simulink model "vhs_fpga_rx_sdram_8k_13xCIC"  (Simulink 7.1)
settings: Solver=FixedStepDiscrete  SolverMode=SingleTasking  StartTime=0.0  StopTime=inf  RelTol=1e-3
undefined symbols (not defined in the file or in its folder): ADC, ADCCIC, ADCClock, BasebandCIC, DAC, Fs, N_frame, N_recv_overlength, VHS
libraries: xbsIndex_r4 x230, vhsadac_common_ob_fpgalib_v1_2_0 x15, misc_tools_fpgalib_v1_0_0 x3, rapid_channel_fpgalib_v1_1_0 x2, misc_tools_dsplib_v1_0_0 x1, sdram_record_playback_fpgalib_v1_0_0 x1, rffe_fpgalib_v1_1_0 x1
(part 1 of 5)
settings Model: Creator=Administrator  LastModifiedBy=lyrtech

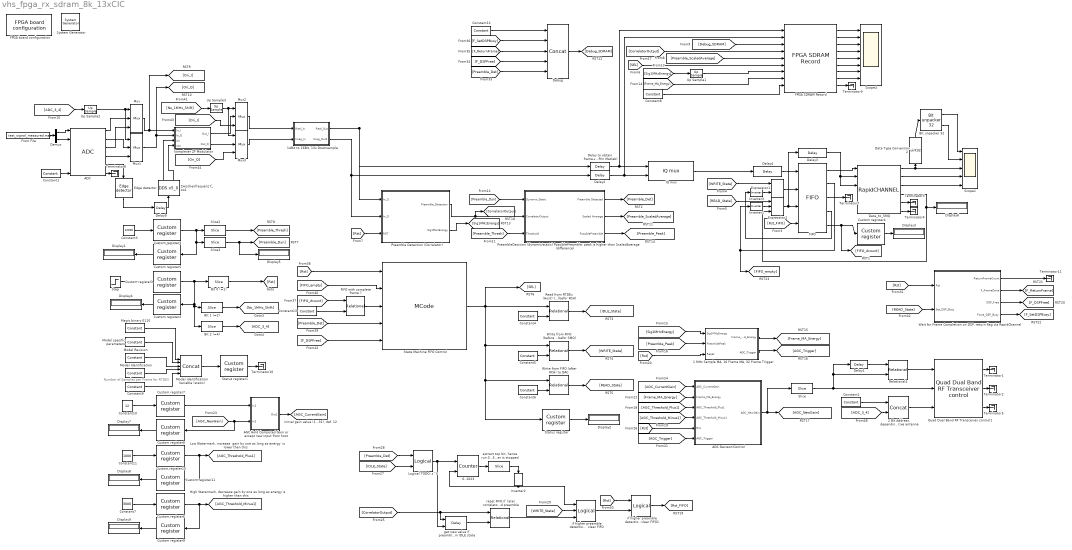
== system vhs_fpga_rx_sdram_8k_13xCIC ==
  note: Number of Samples per Frame for RTDEX
  " System Generator" : xbsIndex_r4/ System Generator  Tag=genX  SystemSampleTime=-1  xilinxfamily=virtex4  part=xc4vsx55  speed=-10  package=ff1148  synthesis_tool=XST  clock_wrapper=Clock Enables  directory=./netlist  testbench=off  simulink_period=1  sysclk_period=9  dcm_input_clock_period=100  incr_netlist=off  trim_vbits=Everywhere in SubSystem  dbl_ovrd=According to Block Masks  core_generation=According to Block Masks  run_coregen=off  deprecated_control=off  eval_field=0  block_type=sysgen
      settings: block_version=10.1.3
  0..1023 : xbsIndex_r4/Counter  cnt_type=Free Running  cnt_to=Inf  operation=Up  start_count=0  cnt_by_val=1  arith_type=Unsigned  n_bits=10  bin_pt=0  load_pin=off  rst=on  en=on  explicit_period=off  period=1  dbl_ovrd=off  use_behavioral_HDL=off  use_rpm=off  implementation=Fabric  block_type=counter
  "1 MHz Sample MA, 16 Frame MA, 32 Frame Trigger" : Subsystem
  "14Bit to 16Bit, 13x Downsample" : Subsystem
  "2 Bit Address, depending on active antenna" : xbsIndex_r4/Concat  num_inputs=2  dbl_ovrd=off  block_type=concat
      settings: block_version=10.1.3
  ADC : vhsadac_common_ob_fpgalib_v1_2_0/ADC  Tag=LYR_FPGA_IO_ADC  Description=Lyrtech block  SystemSampleTime=-1  nbofcha=4  binpt=0  sample_period=ADCClock  ovr_flag=off  trig_sig=on
  AGC Decison/Control : Subsystem
  AGC Hold Computed Gain or accept new input from host : Subsystem
  Bit 0 (=1) : xbsIndex_r4/Slice  nbits=1  boolean_output=on  mode=Lower Bit Location + Width  bit1=-5  base1=MSB of Input  bit0=0  base0=LSB of Input  dbl_ovrd=off  block_type=slice
      settings: infoedit="Extracts a given range of bits from each input sample and presents it at the output.  The output type is ordinarily unsigned with binary point at zero, but can be Boolean when the slice is one bit wide.<P><P>Hardware notes: In hardware this block costs nothing."  block_version=10.1.3
  Bit 1 (=2) : xbsIndex_r4/Slice  nbits=1  boolean_output=off  mode=Lower Bit Location + Width  bit1=-5  base1=MSB of Input  bit0=1  base0=LSB of Input  dbl_ovrd=off  block_type=slice
      settings: infoedit="Extracts a given range of bits from each input sample and presents it at the output.  The output type is ordinarily unsigned with binary point at zero, but can be Boolean when the slice is one bit wide.<P><P>Hardware notes: In hardware this block costs nothing."  block_version=10.1.3
  Bit 2 (=4) : xbsIndex_r4/Slice  nbits=1  boolean_output=off  mode=Lower Bit Location + Width  bit1=-5  base1=MSB of Input  bit0=2  base0=LSB of Input  dbl_ovrd=off  block_type=slice
      settings: infoedit="Extracts a given range of bits from each input sample and presents it at the output.  The output type is ordinarily unsigned with binary point at zero, but can be Boolean when the slice is one bit wide.<P><P>Hardware notes: In hardware this block costs nothing."  block_version=10.1.3
  Bit unpacker 32 : misc_tools_dsplib_v1_0_0/Bit unpacker 32  Tag=LYR_DSP_MISC_BIT_UNPACKER_32  Description=Lyrtech block  output_descriptor=[-16 -16]  data_type=double  frame_size=1
  Constant1 : xbsIndex_r4/Constant  arith_type=Boolean  const=0  n_bits=32  bin_pt=0  explicit_period=on  period=ADCClock  equ=P=C  opselect=C  inp2=PCIN>>17  opr=+  inp1=P  carry=CIN  dbl_ovrd=off  block_type=constant
  Constant10 : Constant  Value=12  OutDataType=sfix(16)  OutScaling=2^0  SampleTime=ADCCIC
  Constant11 : Constant  Value=1000  OutDataType=sfix(16)  OutScaling=2^0  SampleTime=ADCCIC
  Constant12 : xbsIndex_r4/Constant  arith_type=Unsigned  const=0  n_bits=1  bin_pt=0  explicit_period=on  period=ADCCIC  equ=P=C  opselect=C  inp2=PCIN>>17  opr=+  inp1=P  carry=CIN  dbl_ovrd=off  block_type=constant
  Constant13 : xbsIndex_r4/Constant  arith_type=Unsigned  const=N_frame+N_recv_overlength-1  n_bits=16  bin_pt=0  explicit_period=on  period=ADCCIC  equ=P=C  opselect=C  inp2=PCIN>>17  opr=+  inp1=P  carry=CIN  dbl_ovrd=off  block_type=constant
  Constant2 : xbsIndex_r4/Constant  arith_type=Unsigned  const=0  n_bits=1  bin_pt=0  explicit_period=on  period=ADCCIC  equ=P=C  opselect=C  inp2=PCIN>>17  opr=+  inp1=P  carry=CIN  dbl_ovrd=off  block_type=constant
  Constant3 : Constant  Value=12000  OutDataType=sfix(16)  OutScaling=2^0  SampleTime=ADCCIC
  Constant4 : xbsIndex_r4/Constant  arith_type=Unsigned  const=1  n_bits=32  bin_pt=0  explicit_period=on  period=ADCCIC  equ=P=C  opselect=C  inp2=PCIN>>17  opr=+  inp1=P  carry=CIN  dbl_ovrd=off  block_type=constant
  Constant5 : xbsIndex_r4/Constant  arith_type=Unsigned  const=2  n_bits=32  bin_pt=0  explicit_period=on  period=ADCCIC  equ=P=C  opselect=C  inp2=PCIN>>17  opr=+  inp1=P  carry=CIN  dbl_ovrd=off  block_type=constant
  Constant6 : xbsIndex_r4/Constant  arith_type=Unsigned  const=3  n_bits=32  bin_pt=0  explicit_period=on  period=ADCCIC  equ=P=C  opselect=C  inp2=PCIN>>17  opr=+  inp1=P  carry=CIN  dbl_ovrd=off  block_type=constant
  Constant7 : Constant  Value=3000  OutDataType=sfix(16)  OutScaling=2^0  SampleTime=ADCCIC
  Constant8 : xbsIndex_r4/Constant  arith_type=Boolean  const=1  n_bits=32  bin_pt=0  explicit_period=on  period=ADCCIC  equ=P=C  opselect=C  inp2=PCIN>>17  opr=+  inp1=P  carry=CIN  dbl_ovrd=off  block_type=constant
  Constant9 : xbsIndex_r4/Constant  arith_type=Unsigned  const=N_frame+N_recv_overlength  n_bits=15  bin_pt=0  explicit_period=on  period=1  equ=P=C  opselect=C  inp2=PCIN>>17  opr=+  inp1=P  carry=CIN  dbl_ovrd=off  block_type=constant
  Custom register1 : vhsadac_common_ob_fpgalib_v1_2_0/Custom register  Tag=LYR_FPGA_IO_CUSTOM_REGISTER  Description=Lyrtech block  SystemSampleTime=-1  regID=2  direction=Read  output_arithmetic_type=Unsigned  output_width=32  binpt=0  sample_period=ADCCIC
  Custom register10 : vhsadac_common_ob_fpgalib_v1_2_0/Custom register  Tag=LYR_FPGA_IO_CUSTOM_REGISTER  Description=Lyrtech block  SystemSampleTime=-1  regID=5  direction=Read  output_arithmetic_type=Unsigned  output_width=32  binpt=0  sample_period=ADCCIC
  Custom register11 : vhsadac_common_ob_fpgalib_v1_2_0/Custom register  Tag=LYR_FPGA_IO_CUSTOM_REGISTER  Description=Lyrtech block  Orientation=left  SystemSampleTime=-1  regID=5  direction=Write  output_arithmetic_type=Unsigned  output_width=32  binpt=0  sample_period=ADCCIC
  Custom register2 : vhsadac_common_ob_fpgalib_v1_2_0/Custom register  Tag=LYR_FPGA_IO_CUSTOM_REGISTER  Description=Lyrtech block  Orientation=left  SystemSampleTime=-1  regID=2  direction=Write  output_arithmetic_type=Unsigned  output_width=32  binpt=0  sample_period=ADCCIC
  Custom register3 : vhsadac_common_ob_fpgalib_v1_2_0/Custom register  Tag=LYR_FPGA_IO_CUSTOM_REGISTER  Description=Lyrtech block  SystemSampleTime=-1  regID=1  direction=Read  output_arithmetic_type=Unsigned  output_width=32  binpt=0  sample_period=ADCCIC
  Custom register4 : vhsadac_common_ob_fpgalib_v1_2_0/Custom register  Tag=LYR_FPGA_IO_CUSTOM_REGISTER  Description=Lyrtech block  SystemSampleTime=-1  regID=3  direction=Write  output_arithmetic_type=Unsigned  output_width=32  binpt=0  sample_period=ADCCIC
  Custom register5 : vhsadac_common_ob_fpgalib_v1_2_0/Custom register  Tag=LYR_FPGA_IO_CUSTOM_REGISTER  Description=Lyrtech block  Orientation=left  SystemSampleTime=-1  regID=1  direction=Write  output_arithmetic_type=Unsigned  output_width=32  binpt=0  sample_period=ADCCIC
  Custom register6 : vhsadac_common_ob_fpgalib_v1_2_0/Custom register  Tag=LYR_FPGA_IO_CUSTOM_REGISTER  Description=Lyrtech block  SystemSampleTime=-1  regID=6  direction=Read  output_arithmetic_type=Unsigned  output_width=32  binpt=0  sample_period=ADCCIC
  Custom register7 : vhsadac_common_ob_fpgalib_v1_2_0/Custom register  Tag=LYR_FPGA_IO_CUSTOM_REGISTER  Description=Lyrtech block  SystemSampleTime=-1  regID=4  direction=Read  output_arithmetic_type=Unsigned  output_width=32  binpt=0  sample_period=ADCCIC
  Custom register8 : vhsadac_common_ob_fpgalib_v1_2_0/Custom register  Tag=LYR_FPGA_IO_CUSTOM_REGISTER  Description=Lyrtech block  Orientation=left  SystemSampleTime=-1  regID=4  direction=Write  output_arithmetic_type=Unsigned  output_width=32  binpt=0  sample_period=ADCCIC
  Custom register9 : vhsadac_common_ob_fpgalib_v1_2_0/Custom register  Tag=LYR_FPGA_IO_CUSTOM_REGISTER  Description=Lyrtech block  Orientation=left  SystemSampleTime=-1  regID=6  direction=Write  output_arithmetic_type=Unsigned  output_width=32  binpt=0  sample_period=ADCCIC
  Data Type Conversion2 : DataTypeConversion  Orientation=up  OutDataTypeMode=uint32  OutDataType=sfix(16)  OutScaling=2^0  OutDataTypeStr=uint32
  Data_to_SMQ : rapid_channel_fpgalib_v1_1_0/RapidCHANNEL  Tag=LYR_FPGA_IO_RAPIDCHANNEL  Description=Lyrtech block  SystemSampleTime=-1  board_type=VHS-ADC/DAC  interface_quad=LYRIO  interface_drc=LYRIO  interface_dual=LYRIO  direction=TX  output_arithmetic_type=Unsigned  output_width=32  binpt=0  sample_period=ADCCIC  provide_control=on  provide_pio=off  pio1_direction=Input
  Debug : xbsIndex_r4/Concat  num_inputs=5  dbl_ovrd=off  block_type=concat
      settings: block_version=10.1.3
  "Delay to obtain  frame+preamble, note: this is intentionally inaccurate (to enable  preamble detection on DSP/in Matlab)" : xbsIndex_r4/Delay  en=off  latency=690  dbl_ovrd=off  reg_retiming=off  block_type=delay
  Delay{1,3..4,9} (4 alike) : xbsIndex_r4/Delay  en=off  latency=1  dbl_ovrd=off  reg_retiming=off  block_type=delay
      Delay9 settings: xl_area=[200 400 0 400 0 0 0]  block_version=9.2.00
  Delay2 : xbsIndex_r4/Delay  en=off  latency=690  dbl_ovrd=off  reg_retiming=off  block_type=delay
  Demux : Demux  Outputs=2
  Display{1..9} (9 alike) : Display
  Edge detector : misc_tools_fpgalib_v1_0_0/Edge detector  Tag=LYR_FPGA_MISC_EDGE_DETECTOR  Description=Lyrtech block  Orientation=down  SystemSampleTime=-1  edge_detect=Falling  and_latency=0
  Expression1 : xbsIndex_r4/Expression  expression=a & b  align_bp=on  en=off  latency=0  precision=Full  arith_type=Unsigned  n_bits=16  bin_pt=0  dbl_ovrd=off  block_type=expr
      settings: block_version=10.1.3
  Expression2 : xbsIndex_r4/Expression  expression=a & b & c  align_bp=on  en=off  latency=0  precision=Full  arith_type=Unsigned  n_bits=16  bin_pt=0  dbl_ovrd=off  block_type=expr
      settings: block_version=10.1.3
  FIFO : xbsIndex_r4/FIFO  depth=16K  percent_nbits=1  rst=on  en=off  use_dcount=on  use_almost_empty=off  almost_empty_thresh=2  use_almost_full=off  almost_full_thresh=14  dbl_ovrd=off  mem_type=Block RAM  block_type=fifo
      settings: block_version=10.1.3
  "FIFO with complete frame ? " : xbsIndex_r4/Relational  mode=a=b  en=off  latency=0  dbl_ovrd=off  block_type=relational
      settings: block_version=10.1.3
  FPGA board configuration : vhsadac_common_ob_fpgalib_v1_2_0/FPGA board configuration  Tag=SysgenCompile  Description=Lyrtech block  SystemSampleTime=-1  clk_sel=Hardware implementation  clk_src=ADC/DAC clock  hardware=VHS-ADC Virtex-4  copy_bit_cd=on
  FPGA SDRAM Record : sdram_record_playback_fpgalib_v1_0_0/FPGA SDRAM Record  Tag=LYR_FPGA_IO_FPGA_SDRAM_RECORD  Description=Lyrtech block  SystemSampleTime=-1  nbofcha=8  output_arithmetic_type="Signed  (2's comp)"  output_width=16  binpt=0  sample_period=ADCCIC  trig_sig=off
  From File : FromFile  FileName=test_signal_measured.mat  SampleTime=ADCClock
  IQ mux : misc_tools_fpgalib_v1_0_0/IQ mux  Tag=LYR_FPGA_MISC_IQ_MUX  Description=Lyrtech block  SystemSampleTime=-1
  Inverter1 : xbsIndex_r4/Inverter  en=off  latency=0  dbl_ovrd=off  block_type=inv
  Inverter2 : xbsIndex_r4/Inverter  Orientation=down  en=off  latency=0  dbl_ovrd=off  block_type=inv
  Inverter3 : xbsIndex_r4/Inverter  en=off  latency=0  dbl_ovrd=off  block_type=inv
  Logical TODO: z^0 : xbsIndex_r4/Logical  logical_function=AND  inputs=2  en=off  latency=1  precision=Full  arith_type=Unsigned  n_bits=16  bin_pt=0  align_bp=on  dbl_ovrd=off  block_type=logical
  Magic binary 0110 : xbsIndex_r4/Constant  arith_type=Unsigned  const=6  n_bits=4  bin_pt=0  explicit_period=on  period=1  equ=P=C  opselect=C  inp2=PCIN>>17  opr=+  inp1=P  carry=CIN  dbl_ovrd=off  block_type=constant
  Model Identification Variable (static) : xbsIndex_r4/Concat  num_inputs=5  dbl_ovrd=off  block_type=concat
      settings: block_version=10.1.3
  Model Identification : xbsIndex_r4/Constant  arith_type=Unsigned  const=3  n_bits=4  bin_pt=0  explicit_period=on  period=1  equ=P=C  opselect=C  inp2=PCIN>>17  opr=+  inp1=P  carry=CIN  dbl_ovrd=off  block_type=constant
  Model Revision : xbsIndex_r4/Constant  arith_type=Unsigned  const=3  n_bits=3  bin_pt=0  explicit_period=on  period=1  equ=P=C  opselect=C  inp2=PCIN>>17  opr=+  inp1=P  carry=CIN  dbl_ovrd=off  block_type=constant
  Model specific parameters : xbsIndex_r4/Constant  arith_type=Unsigned  const=1  n_bits=6  bin_pt=0  explicit_period=on  period=1  equ=P=C  opselect=C  inp2=PCIN>>17  opr=+  inp1=P  carry=CIN  dbl_ovrd=off  block_type=constant
  Mux{,1..3} (4 alike) : xbsIndex_r4/Mux  inputs=2  en=off  latency=0  precision=Full  arith_type=Unsigned  n_bits=16  bin_pt=14  quantization=Truncate  overflow=Wrap  dbl_ovrd=off  block_type=mux
  Preamble Detection (Correlator) : Subsystem
  PreambleDecision (dynamic/static) PossiblePreamble: peak is higher than ScaledAverage (difference) : Subsystem
  Quad Dual Band RF Transceiver control1 : rffe_fpgalib_v1_1_0/Quad Dual Band RF Transceiver control  Tag=LYR_FPGA_CONTROL_QUAD_DUAL_BAND_RF_TRANSCEIVER_CONTROL  Description=Lyrtech block  SystemSampleTime=-1  external_gain=on  tx1=off  tx2=off  tx3=off  tx4=off  mode=off  add=on  int_divider=off  frac_divider=off  int_divider_en=off  frac_divider_en=off  lock_detect=off  sample_period=ADCCIC
  Read from RTDEx (Host) to FIFO (befor RCH) : xbsIndex_r4/Relational  mode=a=b  en=off  latency=1  dbl_ovrd=off  block_type=relational
      settings: block_version=10.1.3
  Relational4 : xbsIndex_r4/Relational  mode=a!=b  en=off  latency=1  dbl_ovrd=off  block_type=relational
      settings: block_version=10.1.3
  Scope1 : Scope  NumInputPorts=5
      settings: YMin=-5~-5~-5~-5~-5  YMax=5~5~5~5~5  MaxDataPoints=500000
  Scope4 : Scope  NumInputPorts=8
      settings: TimeRange=10  YMin=-5~-5~-5~-5~-5~-5~-5~-5  YMax=5~5~5~5~5~5~5~5  SaveName=ScopeData26  MaxDataPoints=500000
  Slice : xbsIndex_r4/Slice  nbits=7  boolean_output=off  mode=Lower Bit Location + Width  bit1=0  base1=MSB of Input  bit0=0  base0=LSB of Input  dbl_ovrd=off  block_type=slice
      settings: infoedit="Extracts a given range of bits from each input sample and presents it at the output.  The output type is ordinarily unsigned with binary point at zero, but can be Boolean when the slice is one bit wide.<P><P>Hardware notes: In hardware this block costs nothing."  block_version=10.1.3
  Slice2 : xbsIndex_r4/Slice  nbits=31  boolean_output=off  mode=Upper Bit Location + Width  bit1=0  base1=MSB of Input  bit0=0  base0=LSB of Input  dbl_ovrd=off  block_type=slice
      settings: infoedit="Extracts a given range of bits from each input sample and presents it at the output.  The output type is ordinarily unsigned with binary point at zero, but can be Boolean when the slice is one bit wide.<P><P>Hardware notes: In hardware this block costs nothing."  block_version=10.1.3
  Slice3 : xbsIndex_r4/Slice  nbits=1  boolean_output=off  mode=Lower Bit Location + Width  bit1=-5  base1=MSB of Input  bit0=0  base0=LSB of Input  dbl_ovrd=off  block_type=slice
      settings: infoedit="Extracts a given range of bits from each input sample and presents it at the output.  The output type is ordinarily unsigned with binary point at zero, but can be Boolean when the slice is one bit wide.<P><P>Hardware notes: In hardware this block costs nothing."  block_version=10.1.3
  State Machine FIFO Control : xbsIndex_r4/MCode  mfname=vhs_state_machine_fifo  explicit_period=on  period=ADCCIC  inputsTable={'boundInpExpr'=>['','','','',''],'inputs'=>['RST','FIFO_Empty','FIFO_Filled','Preamble_Det','DSPFree']}  outputsTable={'outputs'=>['sel'],'suppressOut'=>['off']}  dbl_ovrd=off  enable_stdout=off  enable_debug=off  suppress_output=1  defparams={}  hide_port_list={}  block_type=mcode
      settings: block_version=10.1.3
  Status register : vhsadac_common_ob_fpgalib_v1_2_0/Custom register  Tag=LYR_FPGA_IO_CUSTOM_REGISTER  Description=Lyrtech block  SystemSampleTime=-1  regID=0  direction=Write  output_arithmetic_type=Unsigned  output_width=32  binpt=0  sample_period=ADCCIC
  Status register1 : vhsadac_common_ob_fpgalib_v1_2_0/Custom register  Tag=LYR_FPGA_IO_CUSTOM_REGISTER  Description=Lyrtech block  SystemSampleTime=-1  regID=7  direction=Write  output_arithmetic_type=Unsigned  output_width=32  binpt=0  sample_period=1
  Step : Step  Time=5  Before=1  After=0  SampleTime=ADCCIC
  Terminator{1..5,7..11} (10 alike) : Terminator
  Up Sample1 : xbsIndex_r4/Up Sample  sample_ratio=BasebandCIC  copy_samples=on  dbl_ovrd=off  block_type=usamp
      settings: infoedit="Up samples input data.  Inserted values  can be zeros or copies of the most recent input sample.<P><P>Hardware notes: No hardware is needed if inserted values are copies of the input sample; otherwise, a mux and single bit flip-flop are used."  block_version=10.1.3
  Up Sample2 : xbsIndex_r4/Up Sample  sample_ratio=ADCCIC  copy_samples=on  dbl_ovrd=off  block_type=usamp
      settings: infoedit="Up samples input data.  Inserted values  can be zeros or copies of the most recent input sample.<P><P>Hardware notes: No hardware is needed if inserted values are copies of the input sample; otherwise, a mux and single bit flip-flop are used."  block_version=10.1.3
  Up Sample3 : xbsIndex_r4/Up Sample  sample_ratio=ADCCIC  copy_samples=on  dbl_ovrd=off  block_type=usamp
      settings: infoedit="Up samples input data.  Inserted values  can be zeros or copies of the most recent input sample.<P><P>Hardware notes: No hardware is needed if inserted values are copies of the input sample; otherwise, a mux and single bit flip-flop are used."  block_version=10.1.3
  "Wait for Frame Completion on DSP, return flag via RapidChannel" : Subsystem
  Write from FIFO (after RCH) to DAC : xbsIndex_r4/Relational  mode=a=b  en=off  latency=1  dbl_ovrd=off  block_type=relational
      settings: block_version=10.1.3
  Write from FIFO (before RCH) to RCH (befor SMQ) : xbsIndex_r4/Relational  mode=a=b  en=off  latency=1  dbl_ovrd=off  block_type=relational
      settings: block_version=10.1.3
  Zwischenfrequenz f_zw1 : xbsIndex_r4/DDS v5_0   Orientation=up  mode=Sine and Cosine  neg_sin=on  neg_cos=off  channels=1  output_frequency_type=Fixed  output_frequency_array=1  phase_offset_type=None  phase_offset_array=[0.0]  channel_port=off  rst=on  en=off  explicit_period=off  period=1  dds_clock_rate=Fs/1e6  sfdr=36.0  frequency_resolution=0.4  acc_latency=One Cycle  noise_shaping=None  dbl_ovrd=off  mem_type=Distributed Memory  pipeline=off  use_rpm=on  block_type=dds
      settings: block_version=9.2.00
  "extract top bit, hence run 0...512 until  the counter is stopped" : xbsIndex_r4/Slice  nbits=31  boolean_output=on  mode=Upper Bit Location + Width  bit1=0  base1=MSB of Input  bit0=0  base0=LSB of Input  dbl_ovrd=off  block_type=slice
      settings: infoedit="Extracts a given range of bits from each input sample and presents it at the output.  The output type is ordinarily unsigned with binary point at zero, but can be Boolean when the slice is one bit wide.<P><P>Hardware notes: In hardware this block costs nothing."  block_version=10.1.3
  get new value if preamble  was detected in IDLE state : xbsIndex_r4/Delay  en=on  latency=1  dbl_ovrd=off  reg_retiming=off  block_type=delay
  "if higher preamble detection value  while in FIFO Write State and  within the last 512 samples since the initially detected preamble,  clear FIFO" : xbsIndex_r4/Logical  logical_function=AND  inputs=3  en=off  latency=0  precision=Full  arith_type=Unsigned  n_bits=16  bin_pt=0  align_bp=on  dbl_ovrd=off  block_type=logical
  "if higher preamble detection value  while in FIFO Write State, clear FIFO1" : xbsIndex_r4/Logical  logical_function=OR  inputs=2  en=off  latency=0  precision=Full  arith_type=Unsigned  n_bits=16  bin_pt=0  align_bp=on  dbl_ovrd=off  block_type=logical
  komplexer ZF Modulator : Subsystem
  reset FIFO if  later correlator output is higher than  initially detected preamble : xbsIndex_r4/Relational  mode=a>b  en=off  latency=1  dbl_ovrd=off  block_type=relational
      settings: block_version=10.1.3
  wires:
  Custom register3/1 -> Slice2/1, Custom register5/1, Slice3/1
  Constant3/1 -> Custom register3/1
  Custom register5/1 -> Display1/1
  Relational4/1 -> Quad Dual Band RF Transceiver control1/1
  Delay1/1 -> Relational4/1
  Slice/1 -> Quad Dual Band RF Transceiver control1/2, Relational4/2, Delay1/1
  Preamble Detection (Correlator)/1(Preamble_Detection) -> PreambleDecision (dynamic/static) PossiblePreamble: peak is higher than ScaledAverage (difference)/2(CorrelatorOutput), [CorrelatorOutput]
  "Delay to obtain  frame+preamble, note: this is intentionally inaccurate (to enable  preamble detection on DSP/in Matlab)"/1 -> IQ mux/1, FPGA SDRAM Record/1
  Delay2/1 -> IQ mux/2, FPGA SDRAM Record/2
  Custom register1/1 -> Custom register2/1, Bit 2 (=4)/1, Bit 1 (=2)/1, Bit 0 (=1)/1
  Step/1 -> Custom register1/1
  IQ mux/1 -> Delay4/1
  FIFO/5 -> Custom register4/1, [FIFO_dcount]
  Custom register4/1 -> Display3/1
  FIFO/1 -> Data_to_SMQ/1
  Constant4/1 -> Read from RTDEx (Host) to FIFO (befor RCH)/2
  Constant5/1 -> Write from FIFO (before RCH) to RCH (befor SMQ)/2
  Read from RTDEx (Host) to FIFO (befor RCH)/1 -> [IDLE_State]
  Write from FIFO (before RCH) to RCH (befor SMQ)/1 -> [WRITE_State]
  Write from FIFO (after RCH) to DAC/1 -> [READ_State]
  Constant6/1 -> Write from FIFO (after RCH) to DAC/2
  Status register/1 -> Display2/1
  State Machine FIFO Control/1 -> Read from RTDEx (Host) to FIFO (befor RCH)/1, Write from FIFO (before RCH) to RCH (befor SMQ)/1, Write from FIFO (after RCH) to DAC/1, Status register/1, [SEL]
  Custom register2/1 -> Display4/1
  [Rst_FIFO] -> FIFO/4
  [WRITE_State] -> Expression1/1
  Expression1/1 -> FIFO/2
  Inverter3/1 -> Expression1/2
  FIFO/4 -> Inverter3/1
  Expression2/1 -> FIFO/3, Delay3/1
  [READ_State] -> Expression2/1
  Inverter1/1 -> Expression2/2
  FIFO/2 -> Inverter1/1, [FIFO_empty]
  Delay3/1 -> Data_to_SMQ/2, Data_to_SMQ/3
  Delay4/1 -> FIFO/1
  Data_to_SMQ/1 -> Data Type Conversion2/1, Scope1/3
  Bit unpacker 32/1 -> Scope1/1
  Bit unpacker 32/2 -> Scope1/2
  Data_to_SMQ/3 -> Scope1/5
  Data_to_SMQ/2 -> Scope1/4
  [Rst] -> Preamble Detection (Correlator)/3(RST)
  Constant8/1 -> FPGA SDRAM Record/9
  FPGA SDRAM Record/8 -> Scope4/8
  FPGA SDRAM Record/7 -> Scope4/7
  FPGA SDRAM Record/6 -> Scope4/6
  FPGA SDRAM Record/5 -> Scope4/5
  FPGA SDRAM Record/4 -> Scope4/4
  FPGA SDRAM Record/3 -> Scope4/3
  FPGA SDRAM Record/2 -> Scope4/2
  FPGA SDRAM Record/1 -> Scope4/1
  [SEL] -> FPGA SDRAM Record/6
  Data_to_SMQ/4 -> Expression2/3, Display6/1
  Mux3/1 -> "14Bit to 16Bit, 13x Downsample"/2(Imag_In)
  Mux2/1 -> "14Bit to 16Bit, 13x Downsample"/1(Real_In)
  "14Bit to 16Bit, 13x Downsample"/1(Real_Out) -> Preamble Detection (Correlator)/1(In_I1), "Delay to obtain  frame+preamble, note: this is intentionally inaccurate (to enable  preamble detection on DSP/in Matlab)"/1
  "14Bit to 16Bit, 13x Downsample"/2(Imag_Out1) -> Preamble Detection (Correlator)/2(In_Q), Delay2/1
  [Preamble_ScaledAverage] -> FPGA SDRAM Record/5
  [Debug_SDRAM] -> FPGA SDRAM Record/3
  Slice2/1 -> [Preamble_Thresh]
  Slice3/1 -> [Preamble_Dyn], Display5/1
  PreambleDecision (dynamic/static) PossiblePreamble: peak is higher than ScaledAverage (difference)/1(Preamble Detected) -> [Preamble_Det]
  [Preamble_Dyn] -> PreambleDecision (dynamic/static) PossiblePreamble: peak is higher than ScaledAverage (difference)/1(Dynamic,Static)
  [Preamble_Thresh] -> PreambleDecision (dynamic/static) PossiblePreamble: peak is higher than ScaledAverage (difference)/3(Threshold)
  [Sig1MHzEnergy] -> Up Sample1/1
  [Frame_MA_Energy] -> FPGA SDRAM Record/8
  Up Sample1/1 -> FPGA SDRAM Record/7
  PreambleDecision (dynamic/static) PossiblePreamble: peak is higher than ScaledAverage (difference)/2(Scaled Average) -> [Preamble_ScaledAverage]
  Model Identification Variable (static)/1 -> Status register1/1
  Constant9/1 -> Model Identification Variable (static)/5
  Model Identification/1 -> Model Identification Variable (static)/4
  Model Revision/1 -> Model Identification Variable (static)/3
  Model specific parameters/1 -> Model Identification Variable (static)/2
  Magic binary 0110/1 -> Model Identification Variable (static)/1
  Preamble Detection (Correlator)/2(Sig1MHzEnergy) -> [Sig1MHzEnergy]
  PreambleDecision (dynamic/static) PossiblePreamble: peak is higher than ScaledAverage (difference)/3(PossiblePreamble) -> [Preamble_Peak]
  Constant10/1 -> Custom register7/1
  Custom register8/1 -> Display7/1
  Custom register10/1 -> Custom register11/1, [AGC_Threshold_Plus1]
  Constant11/1 -> Custom register10/1
  Custom register11/1 -> Display8/1
  Custom register6/1 -> Custom register9/1, [AGC_Threshold_Minus1]
  Constant7/1 -> Custom register6/1
  Custom register9/1 -> Display9/1
  "1 MHz Sample MA, 16 Frame MA, 32 Frame Trigger"/1(Frame_MA_Energy) -> [Frame_MA_Energy]
  Data_to_SMQ/5 -> Terminator3/1
  Data_to_SMQ/6 -> Terminator4/1
  FIFO/3 -> Terminator7/1
  FPGA SDRAM Record/9 -> Terminator9/1
  [Preamble_Peak] -> "1 MHz Sample MA, 16 Frame MA, 32 Frame Trigger"/2(PreamblePeak)
  [Rst] -> "1 MHz Sample MA, 16 Frame MA, 32 Frame Trigger"/3(Reset)
  [AGC_Threshold_Plus1] -> AGC Decison/Control/3(AGC_Threshold_Plus1)
  [AGC_Threshold_Minus1] -> AGC Decison/Control/4(AGC_Threshold_Minus1)
  [AGC_NewGain] -> Custom register8/1, AGC Hold Computed Gain or accept new input from host/2(In2)
  Quad Dual Band RF Transceiver control1/1 -> Terminator1/1
  Quad Dual Band RF Transceiver control1/2 -> Terminator2/1
  Status register1/1 -> Terminator10/1
  Data Type Conversion2/1 -> Bit unpacker 32/1
  [Rst] -> AGC Decison/Control/5(Rst)
  AGC Hold Computed Gain or accept new input from host/1(Out1) -> [AGC_CurrentGain]
  [Sig1MHzEnergy] -> "1 MHz Sample MA, 16 Frame MA, 32 Frame Trigger"/1(Sig1MHzEnergy)
  "1 MHz Sample MA, 16 Frame MA, 32 Frame Trigger"/2(AGC_Trigger) -> [AGC_Trigger]
  [AGC_CurrentGain] -> AGC Decison/Control/1(AGC_CurrentGain)
  [Frame_MA_Energy] -> AGC Decison/Control/2(Frame_MA_Energy)
  AGC Decison/Control/1(AGC_NewGain) -> [AGC_NewGain], Slice/1
  [AGC_Trigger] -> AGC Decison/Control/6(AGC_Trigger)
  Custom register7/1 -> AGC Hold Computed Gain or accept new input from host/1(In1)
  [CorrelatorOutput] -> FPGA SDRAM Record/4
  [Preamble_Det] -> Logical TODO: z^0/1
  [IDLE_State] -> Logical TODO: z^0/2
  Logical TODO: z^0/1 -> 0..1023/1, get new value if preamble  was detected in IDLE state/2
  0..1023/1 -> "extract top bit, hence run 0...512 until  the counter is stopped"/1
  "extract top bit, hence run 0...512 until  the counter is stopped"/1 -> Inverter2/1
  Inverter2/1 -> 0..1023/2, "if higher preamble detection value  while in FIFO Write State and  within the last 512 samples since the initially detected preamble,  clear FIFO"/1
  [CorrelatorOutput] -> get new value if preamble  was detected in IDLE state/1, reset FIFO if  later correlator output is higher than  initially detected preamble/1
  get new value if preamble  was detected in IDLE state/1 -> reset FIFO if  later correlator output is higher than  initially detected preamble/2
  "if higher preamble detection value  while in FIFO Write State and  within the last 512 samples since the initially detected preamble,  clear FIFO"/1 -> "if higher preamble detection value  while in FIFO Write State, clear FIFO1"/2
  [Rst] -> "if higher preamble detection value  while in FIFO Write State, clear FIFO1"/1
  "if higher preamble detection value  while in FIFO Write State, clear FIFO1"/1 -> [Rst_FIFO]
  reset FIFO if  later correlator output is higher than  initially detected preamble/1 -> "if higher preamble detection value  while in FIFO Write State and  within the last 512 samples since the initially detected preamble,  clear FIFO"/3
  [WRITE_State] -> "if higher preamble detection value  while in FIFO Write State and  within the last 512 samples since the initially detected preamble,  clear FIFO"/2
  [READ_State] -> "Wait for Frame Completion on DSP, return flag via RapidChannel"/2(Set_DSP_Busy)
  "Wait for Frame Completion on DSP, return flag via RapidChannel"/3(DSP_Free) -> [F_DSPFree]
  "Wait for Frame Completion on DSP, return flag via RapidChannel"/2(F_FrameDone) -> [F_ReturnFrame]
  "Wait for Frame Completion on DSP, return flag via RapidChannel"/4(Force_DSP_Busy) -> [F_SetDSPBusy]
  [Rst] -> "Wait for Frame Completion on DSP, return flag via RapidChannel"/1(Rst)
  "Wait for Frame Completion on DSP, return flag via RapidChannel"/1(ReturnFrameCount) -> Terminator11/1
  [Preamble_Det] -> Debug/5
  Debug/1 -> [Debug_SDRAM]
  [F_DSPFree] -> Debug/4
  [F_ReturnFrame] -> Debug/3
  [F_SetDSPBusy] -> Debug/2
  Constant12/1 -> Debug/1
  Constant13/1 -> "FIFO with complete frame ? "/2
  [FIFO_dcount] -> "FIFO with complete frame ? "/1
  [Rst] -> State Machine FIFO Control/1
  "FIFO with complete frame ? "/1 -> State Machine FIFO Control/3
  [Preamble_Det] -> State Machine FIFO Control/4
  [FIFO_empty] -> State Machine FIFO Control/2
  [F_DSPFree] -> State Machine FIFO Control/5
  From File/1 -> Demux/1
  Demux/1 -> ADC/1
  Demux/2 -> ADC/2
  Zwischenfrequenz f_zw1/1 -> komplexer ZF Modulator/3(sin)
  Zwischenfrequenz f_zw1/2 -> komplexer ZF Modulator/4(cos)
  Edge detector/1 -> Delay9/1
  Delay9/1 -> Zwischenfrequenz f_zw1/1
  ADC/5 -> Edge detector/1
  ADC/6 -> Terminator8/1
  Constant1/1 -> ADC/6
  Mux/1 -> komplexer ZF Modulator/1(In_I), [Ori_I]
  ADC/3 -> Mux/3
  ADC/1 -> Mux/2
  ADC/2 -> Mux1/2
  ADC/4 -> Mux1/3
  Mux1/1 -> komplexer ZF Modulator/2(In_Q), [Ori_Q]
  [ADC_3_4] -> Up Sample2/1
  [No_1MHz_Shift] -> Up Sample3/1
  komplexer ZF Modulator/2(Out_Q) -> Mux3/2
  komplexer ZF Modulator/1(Out_I) -> Mux2/2
  [Ori_I] -> Mux2/3
  [Ori_Q] -> Mux3/3
  Bit 1 (=2)/1 -> [No_1MHz_Shift]
  Bit 2 (=4)/1 -> [ADC_3_4]
  "2 Bit Address, depending on active antenna"/1 -> Quad Dual Band RF Transceiver control1/3
  Constant2/1 -> "2 Bit Address, depending on active antenna"/1
  [ADC_3_4] -> "2 Bit Address, depending on active antenna"/2
  Quad Dual Band RF Transceiver control1/3 -> Terminator5/1
  Up Sample2/1 -> Mux/1, Mux1/1
  Up Sample3/1 -> Mux2/1, Mux3/1
  Bit 0 (=1)/1 -> [Rst]

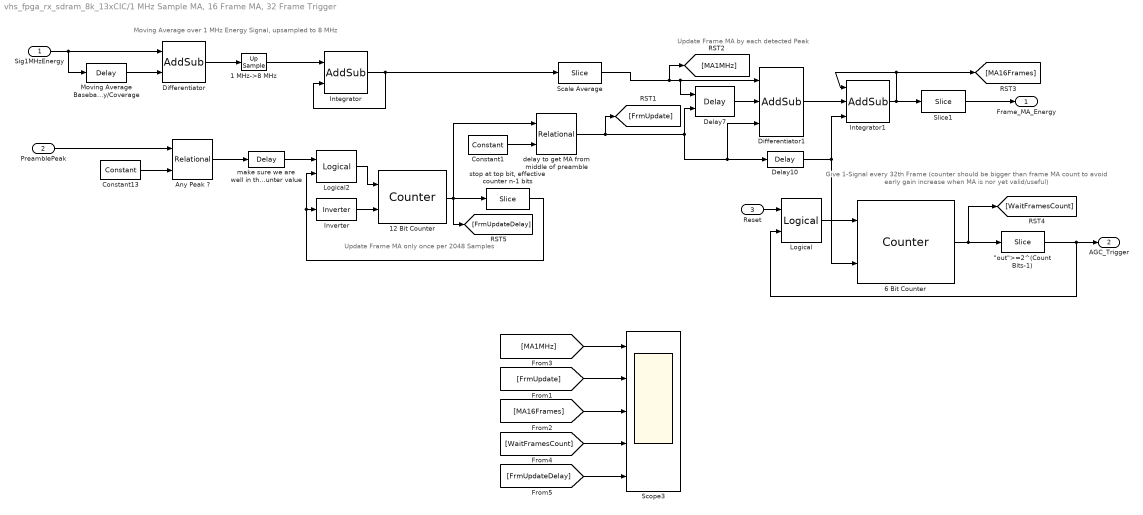
== system vhs_fpga_rx_sdram_8k_13xCIC/1 MHz Sample MA, 16 Frame MA, 32 Frame Trigger ==
  note: Moving Average over 1 MHz Energy Signal, upsampled to 8 MHz
  note: Give 1-Signal every 32th Frame
      | (counter should be bigger than frame MA count to avoid
      | early gain increase when MA is nor yet valid/useful)
  note: Update Frame MA by each detected Peak
  note: Update Frame MA only once per 2048 Samples
  Sig1MHzEnergy : Inport
  PreamblePeak : Inport  Port=2
  Reset : Inport  Port=3
  "\"out\">=2^(Count Bits-1)" : xbsIndex_r4/Slice  nbits=1  boolean_output=on  mode=Upper Bit Location + Width  bit1=0  base1=MSB of Input  bit0=0  base0=LSB of Input  dbl_ovrd=off  block_type=slice
      settings: infoedit="Extracts a given range of bits from each input sample and presents it at the output.  The output type is ordinarily unsigned with binary point at zero, but can be Boolean when the slice is one bit wide.<P><P>Hardware notes: In hardware this block costs nothing."  block_version=10.1.3
  1 MHz->8 MHz : xbsIndex_r4/Up Sample  sample_ratio=BasebandCIC  copy_samples=off  dbl_ovrd=off  block_type=usamp
      settings: infoedit="Up samples input data.  Inserted values  can be zeros or copies of the most recent input sample.<P><P>Hardware notes: No hardware is needed if inserted values are copies of the input sample; otherwise, a mux and single bit flip-flop are used."  block_version=10.1.3
  12 Bit Counter : xbsIndex_r4/Counter  cnt_type=Free Running  cnt_to=Inf  operation=Up  start_count=0  cnt_by_val=1  arith_type=Unsigned  n_bits=12  bin_pt=0  load_pin=off  rst=on  en=on  explicit_period=off  period=1  dbl_ovrd=off  use_behavioral_HDL=off  use_rpm=off  implementation=Fabric  block_type=counter
  6 Bit Counter : xbsIndex_r4/Counter  cnt_type=Free Running  cnt_to=Inf  operation=Up  start_count=0  cnt_by_val=1  arith_type=Unsigned  n_bits=6  bin_pt=0  load_pin=off  rst=on  en=on  explicit_period=off  period=1  dbl_ovrd=off  use_behavioral_HDL=off  use_rpm=off  implementation=Fabric  block_type=counter
  Any Peak ? : xbsIndex_r4/Relational  mode=a>=b  en=off  latency=1  dbl_ovrd=off  block_type=relational
      settings: block_version=10.1.3
  Constant1 : xbsIndex_r4/Constant  arith_type=Unsigned  const=512  n_bits=12  bin_pt=0  explicit_period=on  period=ADCCIC  equ=P=C  opselect=C  inp2=PCIN>>17  opr=+  inp1=P  carry=CIN  dbl_ovrd=off  block_type=constant
  Constant13 : xbsIndex_r4/Constant  arith_type=Unsigned  const=3  n_bits=16  bin_pt=0  explicit_period=on  period=ADCCIC  equ=P=C  opselect=C  inp2=PCIN>>17  opr=+  inp1=P  carry=CIN  dbl_ovrd=off  block_type=constant
  Delay10 : xbsIndex_r4/Delay  en=off  latency=1  dbl_ovrd=off  reg_retiming=off  block_type=delay
  Delay7 : xbsIndex_r4/Delay  en=on  latency=16  dbl_ovrd=off  reg_retiming=off  block_type=delay
  Differentiator : xbsIndex_r4/AddSub  mode=Subtraction  use_carryin=off  use_carryout=off  en=off  latency=0  precision=Full  arith_type=Unsigned  n_bits=16  bin_pt=14  quantization=Truncate  overflow=Wrap  dbl_ovrd=off  use_behavioral_HDL=off  pipelined=off  use_rpm=on  hw_selection=Fabric  block_type=addsub
      settings: block_version=10.1.3
  Differentiator1 : xbsIndex_r4/AddSub  mode=Subtraction  use_carryin=off  use_carryout=off  en=on  latency=1  precision=Full  arith_type=Unsigned  n_bits=16  bin_pt=14  quantization=Truncate  overflow=Wrap  dbl_ovrd=off  use_behavioral_HDL=off  pipelined=off  use_rpm=on  hw_selection=Fabric  block_type=addsub
      settings: block_version=10.1.3
  Integrator : xbsIndex_r4/AddSub  mode=Addition  use_carryin=off  use_carryout=off  en=off  latency=1  precision=User Defined  arith_type="Signed  (2's comp)"  n_bits=22  bin_pt=0  quantization=Truncate  overflow=Saturate  dbl_ovrd=off  use_behavioral_HDL=off  pipelined=off  use_rpm=on  hw_selection=Fabric  block_type=addsub
      settings: block_version=10.1.3
  Integrator1 : xbsIndex_r4/AddSub  mode=Addition  use_carryin=off  use_carryout=off  en=on  latency=1  precision=User Defined  arith_type="Signed  (2's comp)"  n_bits=21  bin_pt=0  quantization=Truncate  overflow=Saturate  dbl_ovrd=off  use_behavioral_HDL=off  pipelined=off  use_rpm=on  hw_selection=Fabric  block_type=addsub
      settings: block_version=10.1.3
  Inverter : xbsIndex_r4/Inverter  en=off  latency=0  dbl_ovrd=off  block_type=inv
  Logical : xbsIndex_r4/Logical  logical_function=OR  inputs=2  en=off  latency=0  precision=Full  arith_type=Unsigned  n_bits=16  bin_pt=0  align_bp=on  dbl_ovrd=off  block_type=logical
  Logical2 : xbsIndex_r4/Logical  logical_function=AND  inputs=2  en=off  latency=0  precision=Full  arith_type=Unsigned  n_bits=16  bin_pt=0  align_bp=on  dbl_ovrd=off  block_type=logical
  Moving Average Baseband (1MHz) Delay/Coverage : xbsIndex_r4/Delay  en=off  latency=40  dbl_ovrd=off  reg_retiming=off  block_type=delay
  Scale Average : xbsIndex_r4/Slice  nbits=16  boolean_output=off  mode=Upper Bit Location + Width  bit1=0  base1=MSB of Input  bit0=0  base0=LSB of Input  dbl_ovrd=off  block_type=slice
      settings: infoedit="Extracts a given range of bits from each input sample and presents it at the output.  The output type is ordinarily unsigned with binary point at zero, but can be Boolean when the slice is one bit wide.<P><P>Hardware notes: In hardware this block costs nothing."  block_version=10.1.3
  Scope3 : Scope  NumInputPorts=5
      settings: TimeRange=10  YMin=4.75~-9.45~2297~-1155~-5  YMax=5.25~-8.55~2306~-1151~5  SaveName=ScopeData6  MaxDataPoints=500000
  Slice1 : xbsIndex_r4/Slice  nbits=16  boolean_output=off  mode=Upper Bit Location + Width  bit1=0  base1=MSB of Input  bit0=0  base0=LSB of Input  dbl_ovrd=off  block_type=slice
      settings: infoedit="Extracts a given range of bits from each input sample and presents it at the output.  The output type is ordinarily unsigned with binary point at zero, but can be Boolean when the slice is one bit wide.<P><P>Hardware notes: In hardware this block costs nothing."  block_version=10.1.3
  delay to get MA from middle of preamble : xbsIndex_r4/Relational  mode=a=b  en=off  latency=1  dbl_ovrd=off  block_type=relational
      settings: block_version=10.1.3
  "make sure we are  well in the preamble when updating frame energy MA (416 for 13 MHz system, here *8/13=256) -> delay logic moved to more efficient comparison  with counter value" : xbsIndex_r4/Delay  en=off  latency=1  dbl_ovrd=off  reg_retiming=off  block_type=delay
  "stop at top bit, effective counter n-1 bits" : xbsIndex_r4/Slice  nbits=1  boolean_output=on  mode=Upper Bit Location + Width  bit1=0  base1=MSB of Input  bit0=0  base0=LSB of Input  dbl_ovrd=off  block_type=slice
      settings: infoedit="Extracts a given range of bits from each input sample and presents it at the output.  The output type is ordinarily unsigned with binary point at zero, but can be Boolean when the slice is one bit wide.<P><P>Hardware notes: In hardware this block costs nothing."  block_version=10.1.3
  Frame_MA_Energy : Outport
  AGC_Trigger : Outport  Port=2
  wires:
  Moving Average Baseband (1MHz) Delay/Coverage/1 -> Differentiator/2
  Differentiator/1 -> 1 MHz->8 MHz/1
  Integrator/1 -> Integrator/2, Scale Average/1
  Sig1MHzEnergy/1 -> Moving Average Baseband (1MHz) Delay/Coverage/1, Differentiator/1
  1 MHz->8 MHz/1 -> Integrator/1
  Delay7/1 -> Differentiator1/2
  Scale Average/1 -> Delay7/1, Differentiator1/1, [MA1MHz]
  Delay10/1 -> Integrator1/3, 6 Bit Counter/2
  Differentiator1/1 -> Integrator1/2
  Integrator1/1 -> Slice1/1, Integrator1/1, [MA16Frames]
  Any Peak ?/1 -> "make sure we are  well in the preamble when updating frame energy MA (416 for 13 MHz system, here *8/13=256) -> delay logic moved to more efficient comparison  with counter value"/1
  Constant13/1 -> Any Peak ?/2
  6 Bit Counter/1 -> "\"out\">=2^(Count Bits-1)"/1, [WaitFramesCount]
  "\"out\">=2^(Count Bits-1)"/1 -> Logical/2, AGC_Trigger/1
  Logical/1 -> 6 Bit Counter/1
  12 Bit Counter/1 -> "stop at top bit, effective counter n-1 bits"/1, [FrmUpdateDelay], delay to get MA from middle of preamble/1
  "stop at top bit, effective counter n-1 bits"/1 -> Inverter/1, Logical2/2
  Inverter/1 -> 12 Bit Counter/2
  Logical2/1 -> 12 Bit Counter/1
  "make sure we are  well in the preamble when updating frame energy MA (416 for 13 MHz system, here *8/13=256) -> delay logic moved to more efficient comparison  with counter value"/1 -> Logical2/1
  Slice1/1 -> Frame_MA_Energy/1
  PreamblePeak/1 -> Any Peak ?/1
  Reset/1 -> Logical/1
  [MA1MHz] -> Scope3/1
  [FrmUpdate] -> Scope3/2
  [MA16Frames] -> Scope3/3
  [WaitFramesCount] -> Scope3/4
  [FrmUpdateDelay] -> Scope3/5
  delay to get MA from middle of preamble/1 -> Delay10/1, Differentiator1/3, Delay7/2, [FrmUpdate]
  Constant1/1 -> delay to get MA from middle of preamble/2
